simulink model "TDMA"  (R2022b)
settings: Solver=VariableStepAuto  StartTime=0.0  StopTime=10.0  RelTol=1e-3
libraries: dsparch4 x4
settings Model: Creator=Admin  LastModifiedBy=Admin

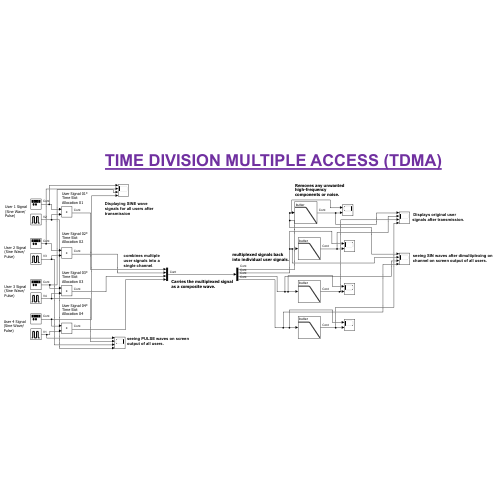
[thumbnail: Simulink's stored preview of the top-level diagram]
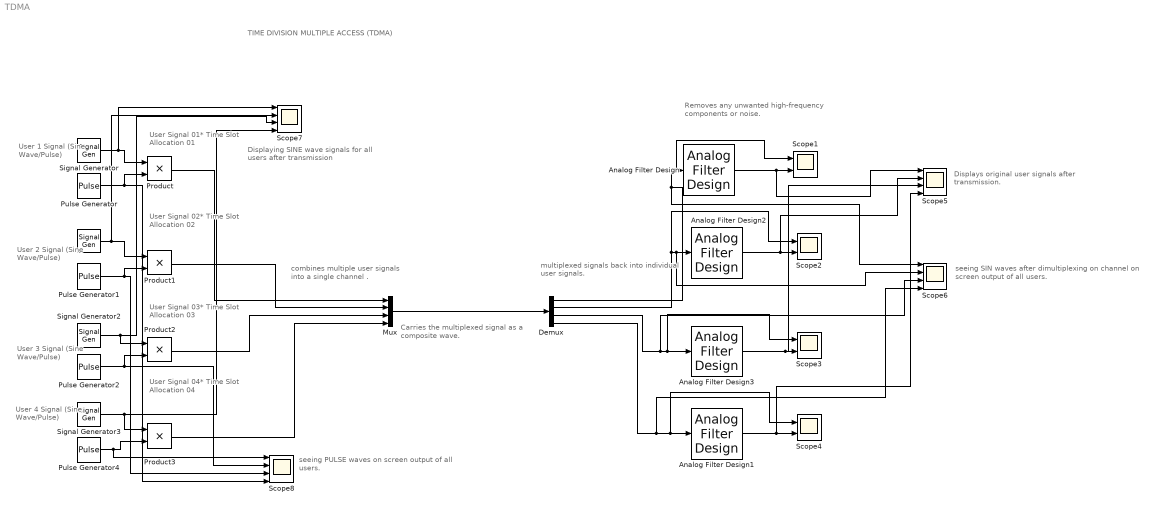
== system TDMA ==
  note: User Signal 01* Time Slot Allocation 01
  note: User 3 Signal (Sine Wave/Pulse)
  note: User 4 Signal (Sine Wave/Pulse)
  note: User 2 Signal (Sine Wave/Pulse)
  note: User 1 Signal (Sine Wave/Pulse)
  note: Removes any unwanted high-frequency components or noise.
  note: multiplexed signals back into individual user signals.
  note: Carries the multiplexed signal as a composite wave.
  note: combines multiple user signals into a single channel .
  note: seeing SIN waves after dimultiplexing on channel on screen output of all users.
  note: Displays original user signals after transmission.
  note: seeing PULSE waves on screen output of all users.
  note: TIME DIVISION MULTIPLE ACCESS (TDMA)
  note: Displaying SINE wave signals for all users after transmission
  note: User Signal 02* Time Slot Allocation 02
  note: User Signal 03* Time Slot Allocation 03
  note: User Signal 04* Time Slot Allocation 04
  " " : SignalGenerator  Amplitude=4  Frequency=3*pi  Units=rad/sec
  Analog Filter Design{,1..3} (4 alike) : dsparch4/Analog Filter Design  method=Butterworth  filttype=Lowpass  N=8  Wlo=30  Whi=80  Rp=2  Rs=40
  Demux : Demux
  Mux : Mux
  Product{,1..3} (4 alike) : Product
  Pulse Generator : DiscretePulseGenerator  PulseType=Time based  Period=0.1  PulseWidth=25  PhaseDelay=0.1
  Pulse Generator1 : DiscretePulseGenerator  PulseType=Time based  Period=0.1  PulseWidth=25  PhaseDelay=0.01
  Pulse Generator2 : DiscretePulseGenerator  PulseType=Time based  Period=0.1  PulseWidth=25  PhaseDelay=0.001
  Pulse Generator4 : DiscretePulseGenerator  PulseType=Time based  Period=0.1  PulseWidth=25  PhaseDelay=0.0001
  Scope{1..4} (4 alike) : Scope  NumInputPorts=2
  Scope{5..8} (4 alike) : Scope  NumInputPorts=4
  Signal Generator : SignalGenerator  Amplitude=4  Frequency=2*pi  Units=rad/sec
  Signal Generator2 : SignalGenerator  Amplitude=4  Frequency=4*pi  Units=rad/sec
  Signal Generator3 : SignalGenerator  Amplitude=4  Frequency=5*pi  Units=rad/sec
  wires:
  Product/1 -> Mux/1
  Product1/1 -> Mux/2
  Product2/1 -> Mux/3
  Product3/1 -> Mux/4
  Mux/1 -> Demux/1
  Signal Generator/1 -> Scope7/1, Product/1
  Pulse Generator/1 -> Scope8/4, Product/2
  " "/1 -> Scope7/2, Product1/1
  Pulse Generator1/1 -> Scope8/3, Product1/2
  Signal Generator2/1 -> Scope7/3, Product2/1
  Pulse Generator2/1 -> Scope8/2, Product2/2
  Signal Generator3/1 -> Scope7/4, Product3/1
  Pulse Generator4/1 -> Scope8/1, Product3/2
  Demux/1 -> Scope1/1, Analog Filter Design/1, Scope6/1
  Demux/2 -> Scope2/1, Scope6/2, Analog Filter Design2/1
  Demux/3 -> Scope6/3, Scope3/1, Analog Filter Design3/1
  Demux/4 -> Scope6/4, Scope4/1, Analog Filter Design1/1
  Analog Filter Design/1 -> Scope5/1, Scope1/2
  Analog Filter Design2/1 -> Scope5/2, Scope2/2
  Analog Filter Design3/1 -> Scope5/3, Scope3/2
  Analog Filter Design1/1 -> Scope5/4, Scope4/2
